simulink model "blovtb"  (Simulink 8.5)
settings: Solver=ode45  SolverMode=SingleTasking  StartTime=0.0  StopTime=6  MaxStep=.002  RelTol=1e-3  AbsTol=1e-6
settings Model: Creator=PC  LastModifiedBy=PC  ExtModeTrigMode=oneshot  ExtModeArmWhenConnect=off
settings DataIOCC: LimitDataPoints=off
settings OptimizationCC: BlockReduction=off  BooleanDataType=off  ExpressionDepthLimit=128
settings DebuggingCC: SaveWithParameterizedLinksMsg=none  SignalResolutionControl=TryResolveAllWithWarning  MultiTaskDSMMsg=warning  MultiTaskCondExecSysMsg=none  FcnCallInpInsideContextMsg=EnableAllAsError  StateNameClashWarn=none  StrictBusMsg=None
settings HardwareCC: TargetUnknown=on

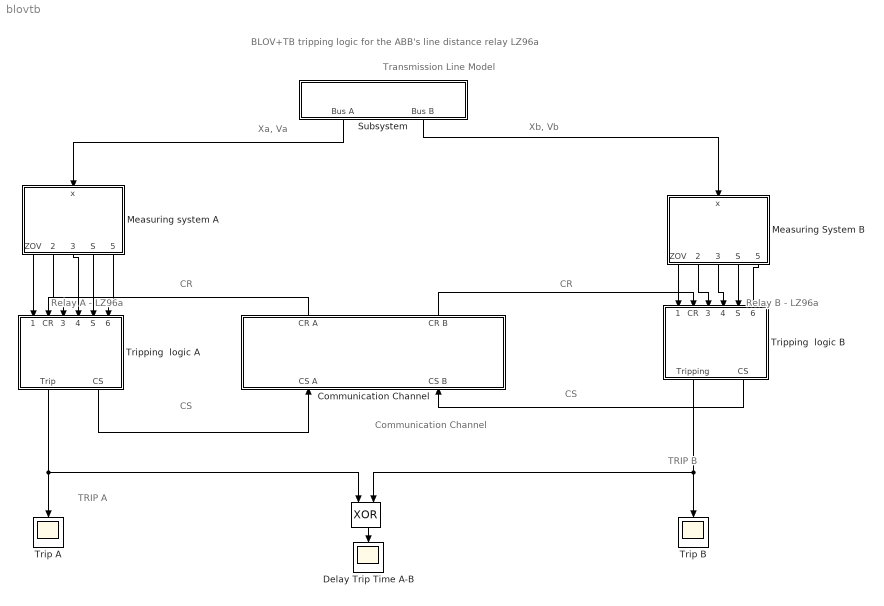
== system blovtb ==
  note: Transmission Line Model
  note: Relay A - LZ96a
  note: Xa, Va
  note: Xb, Vb
  note: CS
  note: CS
  note: CR
  note: CR
  note: TRIP A
  note: TRIP B
  note: Relay B - LZ96a
  note: Communication
      | Channel
  note: BLOV+TB tripping logic for the ABB's line distance relay LZ96a
  " " : Logic  Operator=XOR
  Communication Channel : Subsystem  mask(Communication channel.){Tdelay=0, failureA=on, failureB=on, err_signal=0}
      mask prompts: Tdelay "Channel delay time [ms]:"; failureA "A to B Communication channel failure."; failureB "B to A Communication Channel failure"; err_signal "Erroneous signal:"
      mask TypeOptions err_signal: 0 | 1
  Delay Trip Time A-B : Scope
      settings: TickLabels=on  YMin=-0.5  YMax=2
  Measuring System B : Subsystem  mask(Measuring system - starter block){ZM=[0 1.8 2.5], Tzone=[0 0.4 0.6], S=[-1 3], Tstarter=0.8, ZOV=1.3, ZMB=-1.3, tHF1=0.2}
      mask prompts: ZM "Zone reach [z1 z2  z3]  [p.u.]:"; Tzone "Zone times [z1 z2  z3]  [s]:"; S "Starter range [Smin Smax] [p.u.]:"; Tstarter "Starter time [s]:"; ZOV "ZOV (pu)"; ZMB "ZMB (p.u.):"; tHF1 "tHF(s)"
      mask init:
      | SB=S(1);
      | SF=S(2);
      | t4=Tstarter;
      | ZM1=ZM(1);
      | ZM2=ZM(2);
      | ZM3=ZM(3);
      | t1=Tzone(1);
      | t2=Tzone(2);
      | t3=Tzone(3);
  Measuring system A : Subsystem  mask(Measuring system - starter block){ZM=[0 1.8 2.5], Tzone=[0 0.4 0.6], S=[-1 4], Tstarter=0.8, ZOV=1.3, ZMB=-1.3, tHF1=0.2}
      mask prompts: ZM "Zone reach [z1 z2  z3]  [p.u.]:"; Tzone "Zone times [z1 z2  z3]  [s]:"; S "Starter range [Smin Smax] [p.u.]:"; Tstarter "Starter time [s]:"; ZOV "ZOV (pu)"; ZMB "ZMB (p.u.):"; tHF1 "tHF(s)"
      mask init:
      | SB=S(1);
      | SF=S(2);
      | t4=Tstarter;
      | ZM1=ZM(1);
      | ZM2=ZM(2);
      | ZM3=ZM(3);
      | t1=Tzone(1);
      | t2=Tzone(2);
      | t3=Tzone(3);
  Subsystem : Subsystem  mask(Model of transmission line with fault){x=1.1, Tfault=1}
      mask prompts: x "Fault location from bus A [p.u.]"; Tfault "Fault time [s]:"
  Trip A : Scope
      settings: TickLabels=on  YMin=-0.5  YMax=2
  Trip B : Scope
      settings: TickLabels=on  YMin=-0.5  YMax=2
  Tripping  logic A : Subsystem
  Tripping  logic B : Subsystem
  wires:
  " "/1 -> Delay Trip Time A-B/1
  Measuring system A/4(S) -> Tripping  logic A/5(S)
  Measuring system A/3(ZM3 Output) -> Tripping  logic A/4(ZM3)
  Measuring system A/5(ZMB) -> Tripping  logic A/6(ZMB)
  Subsystem/1(Bus A) -> Measuring system A/1(x)
  Tripping  logic A/2(CS) -> Communication Channel/1(CS A)
  Communication Channel/1(CR A) -> Tripping  logic A/2(CR)
  Measuring System B/4(S) -> Tripping  logic B/5(S)
  Measuring System B/3(ZM3 Output) -> Tripping  logic B/4(ZM3)
  Measuring System B/2(ZM2 Output) -> Tripping  logic B/3(ZM2)
  Measuring System B/5(ZMB) -> Tripping  logic B/6(ZMB)
  Measuring System B/1(ZOV) -> Tripping  logic B/1(ZOV)
  Subsystem/2(Bus B) -> Measuring System B/1(x)
  Tripping  logic B/1(Tripping) -> Trip B/1, " "/2
  Tripping  logic B/2(CS) -> Communication Channel/2(CS B)
  Communication Channel/2(CR B) -> Tripping  logic B/2(CR)
  Tripping  logic A/1(Trip) -> Trip A/1, " "/1
  Measuring system A/1(ZOV) -> Tripping  logic A/1(ZOV)
  Measuring system A/2(ZM2 Output) -> Tripping  logic A/3(ZM2)

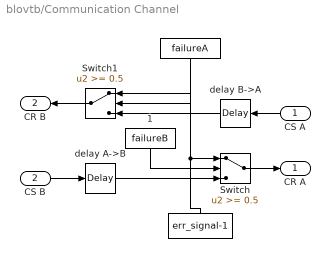
== system blovtb/Communication Channel ==
  CS A : Inport
  CS B : Inport  Port=2
  " " : Constant  Value=failureA
  "  " : Constant  Value=err_signal-1
  " 1" : Constant  Value=failureB
  Switch : Switch  Threshold=0.5  SaturateOnIntegerOverflow=on  InputSameDT=on
  Switch1 : Switch  Threshold=0.5  SaturateOnIntegerOverflow=on  InputSameDT=on
  delay A->B : TransportDelay  DelayTime=Tdelay/1000+1e-12
  delay B->A : TransportDelay  DelayTime=Tdelay/1000+1e-12
  CR A : Outport  InitialOutput=0
  CR B : Outport  Port=2  InitialOutput=0
  wires:
  Switch/1 -> CR A/1
  CS B/1 -> delay A->B/1
  CS A/1 -> delay B->A/1
  Switch1/1 -> CR B/1
  "  "/1 -> Switch1/1, Switch/1
  delay A->B/1 -> Switch/3
  delay B->A/1 -> Switch1/3
  " "/1 -> Switch1/2
  " 1"/1 -> Switch/2

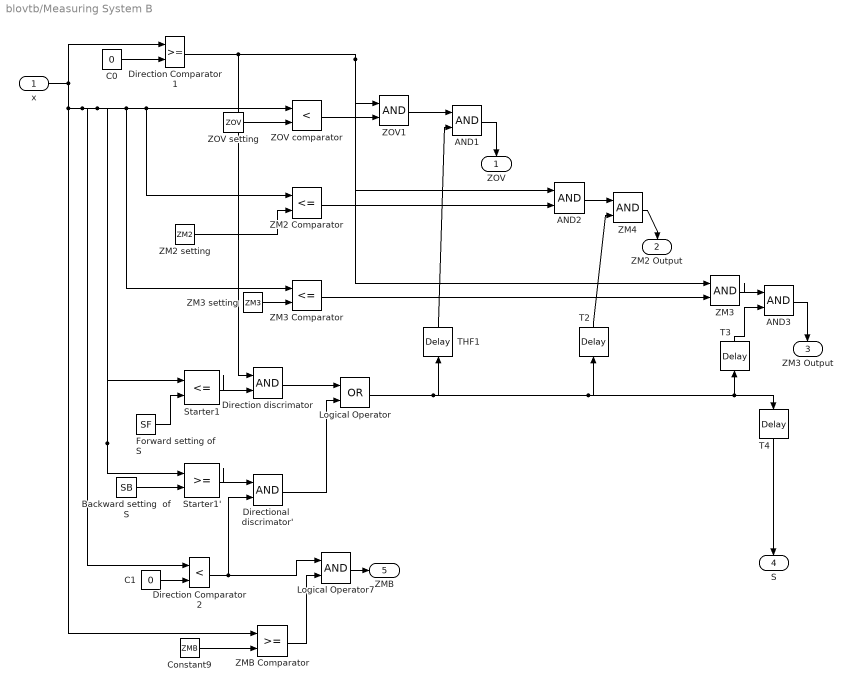
== system blovtb/Measuring System B ==
  x : Inport
  AND1 : Logic
  AND2 : Logic
  AND3 : Logic
  Backward setting  of S : Constant  Value=SB
  C0 : Constant  Value=0
  C1 : Constant  Value=0
  Constant9 : Constant  Value=ZMB
  Direction Comparator1 : RelationalOperator  InputSameDT=on
  Direction Comparator2 : RelationalOperator  Operator=<  InputSameDT=on
  Direction discrimator : Logic
  Directional  discrimator' : Logic
  Forward setting of S : Constant  Value=SF
  Logical Operator : Logic  Operator=OR
  Logical Operator7 : Logic
  Starter1 : RelationalOperator  Operator=<=  InputSameDT=on
  Starter1' : RelationalOperator  InputSameDT=on
  T2 : TransportDelay  DelayTime=t2
  T3 : TransportDelay  DelayTime=t3
  T4 : TransportDelay  DelayTime=t4
  THF1 : TransportDelay  DelayTime=tHF1
  ZM2 Comparator : RelationalOperator  Operator=<=  InputSameDT=on
  ZM2 setting : Constant  Value=ZM2
  ZM3 : Logic
  ZM3 Comparator : RelationalOperator  Operator=<=  InputSameDT=on
  ZM3 setting : Constant  Value=ZM3
  ZM4 : Logic
  ZMB Comparator : RelationalOperator  InputSameDT=on
  ZOV comparator : RelationalOperator  Operator=<  InputSameDT=on
  ZOV setting : Constant  Value=ZOV
  ZOV1 : Logic
  ZOV : Outport  InitialOutput=0
  ZM2 Output : Outport  Port=2  InitialOutput=0
  ZM3 Output : Outport  Port=3  InitialOutput=0
  S : Outport  Port=4  InitialOutput=0
  ZMB : Outport  Port=5  InitialOutput=0
  wires:
  ZM2 setting/1 -> ZM2 Comparator/2
  C0/1 -> Direction Comparator1/2
  x/1 -> Direction Comparator1/1, ZM2 Comparator/1, ZOV comparator/1, ZM3 Comparator/1, Starter1/1, Starter1'/1, Direction Comparator2/1, ZMB Comparator/1
  Forward setting of S/1 -> Starter1/2
  Constant9/1 -> ZMB Comparator/2
  ZMB Comparator/1 -> Logical Operator7/2
  C1/1 -> Direction Comparator2/2
  Logical Operator7/1 -> ZMB/1
  ZM3 Comparator/1 -> ZM3/2
  ZM2 Comparator/1 -> AND2/2
  AND2/1 -> ZM4/1
  ZM3/1 -> AND3/1
  Backward setting  of S/1 -> Starter1'/2
  T4/1 -> S/1
  T2/1 -> ZM4/2
  ZM4/1 -> ZM2 Output/1
  T3/1 -> AND3/2
  AND3/1 -> ZM3 Output/1
  Starter1/1 -> Direction discrimator/2
  Direction Comparator1/1 -> ZOV1/1, AND2/1, ZM3/1, Direction discrimator/1
  Direction discrimator/1 -> Logical Operator/1
  Starter1'/1 -> Directional  discrimator'/1
  Directional  discrimator'/1 -> Logical Operator/2
  Logical Operator/1 -> THF1/1, T2/1, T4/1, T3/1
  Direction Comparator2/1 -> Logical Operator7/1, Directional  discrimator'/2
  ZM3 setting/1 -> ZM3 Comparator/2
  ZOV setting/1 -> ZOV comparator/2
  ZOV comparator/1 -> ZOV1/2
  ZOV1/1 -> AND1/1
  THF1/1 -> AND1/2
  AND1/1 -> ZOV/1

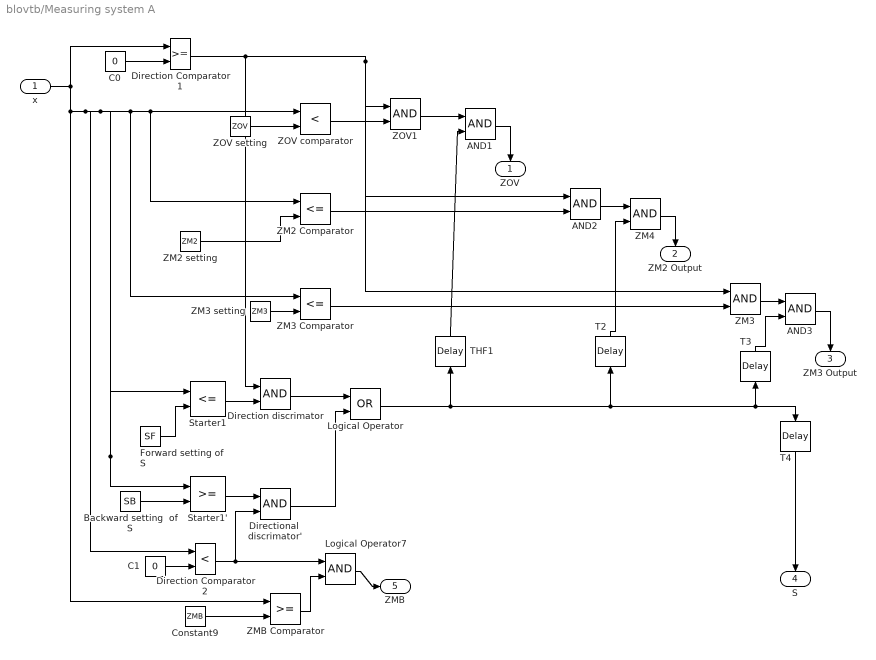
== system blovtb/Measuring system A ==
  x : Inport
  AND1 : Logic
  AND2 : Logic
  AND3 : Logic
  Backward setting  of S : Constant  Value=SB
  C0 : Constant  Value=0
  C1 : Constant  Value=0
  Constant9 : Constant  Value=ZMB
  Direction Comparator1 : RelationalOperator  InputSameDT=on
  Direction Comparator2 : RelationalOperator  Operator=<  InputSameDT=on
  Direction discrimator : Logic
  Directional  discrimator' : Logic
  Forward setting of S : Constant  Value=SF
  Logical Operator : Logic  Operator=OR
  Logical Operator7 : Logic
  Starter1 : RelationalOperator  Operator=<=  InputSameDT=on
  Starter1' : RelationalOperator  InputSameDT=on
  T2 : TransportDelay  DelayTime=t2
  T3 : TransportDelay  DelayTime=t3
  T4 : TransportDelay  DelayTime=t4
  THF1 : TransportDelay  DelayTime=tHF1
  ZM2 Comparator : RelationalOperator  Operator=<=  InputSameDT=on
  ZM2 setting : Constant  Value=ZM2
  ZM3 : Logic
  ZM3 Comparator : RelationalOperator  Operator=<=  InputSameDT=on
  ZM3 setting : Constant  Value=ZM3
  ZM4 : Logic
  ZMB Comparator : RelationalOperator  InputSameDT=on
  ZOV comparator : RelationalOperator  Operator=<  InputSameDT=on
  ZOV setting : Constant  Value=ZOV
  ZOV1 : Logic
  ZOV : Outport  InitialOutput=0
  ZM2 Output : Outport  Port=2  InitialOutput=0
  ZM3 Output : Outport  Port=3  InitialOutput=0
  S : Outport  Port=4  InitialOutput=0
  ZMB : Outport  Port=5  InitialOutput=0
  wires:
  ZM2 setting/1 -> ZM2 Comparator/2
  C0/1 -> Direction Comparator1/2
  x/1 -> Direction Comparator1/1, ZM2 Comparator/1, ZOV comparator/1, ZM3 Comparator/1, Starter1/1, Starter1'/1, Direction Comparator2/1, ZMB Comparator/1
  Forward setting of S/1 -> Starter1/2
  Constant9/1 -> ZMB Comparator/2
  ZMB Comparator/1 -> Logical Operator7/2
  C1/1 -> Direction Comparator2/2
  Logical Operator7/1 -> ZMB/1
  ZM3 Comparator/1 -> ZM3/2
  ZM2 Comparator/1 -> AND2/2
  AND2/1 -> ZM4/1
  ZM3/1 -> AND3/1
  Backward setting  of S/1 -> Starter1'/2
  T4/1 -> S/1
  T2/1 -> ZM4/2
  ZM4/1 -> ZM2 Output/1
  T3/1 -> AND3/2
  AND3/1 -> ZM3 Output/1
  Starter1/1 -> Direction discrimator/2
  Direction Comparator1/1 -> ZOV1/1, AND2/1, ZM3/1, Direction discrimator/1
  Direction discrimator/1 -> Logical Operator/1
  Starter1'/1 -> Directional  discrimator'/1
  Directional  discrimator'/1 -> Logical Operator/2
  Logical Operator/1 -> THF1/1, T2/1, T4/1, T3/1
  Direction Comparator2/1 -> Logical Operator7/1, Directional  discrimator'/2
  ZM3 setting/1 -> ZM3 Comparator/2
  ZOV setting/1 -> ZOV comparator/2
  ZOV comparator/1 -> ZOV1/2
  ZOV1/1 -> AND1/1
  THF1/1 -> AND1/2
  AND1/1 -> ZOV/1

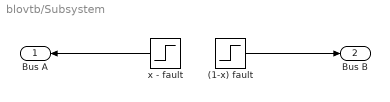
== system blovtb/Subsystem ==
  (1-x) fault : Step  Time=Tfault  Before=1000  After=1-x  SampleTime=0
  x - fault : Step  Time=Tfault  Before=1000  After=x  SampleTime=0
  Bus A : Outport  InitialOutput=0
  Bus B : Outport  Port=2  InitialOutput=0
  wires:
  x - fault/1 -> Bus A/1
  (1-x) fault/1 -> Bus B/1

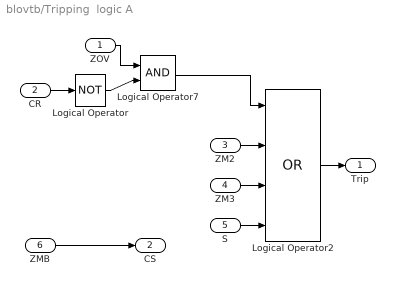
== system blovtb/Tripping  logic A ==
  ZOV : Inport
  CR : Inport  Port=2
  ZM2 : Inport  Port=3
  ZM3 : Inport  Port=4
  S : Inport  Port=5
  ZMB : Inport  Port=6
  Logical Operator : Logic  Operator=NOT  Inputs=1
  Logical Operator2 : Logic  Operator=OR  Inputs=4
  Logical Operator7 : Logic
  Trip : Outport  InitialOutput=0
  CS : Outport  Port=2  InitialOutput=0
  wires:
  ZMB/1 -> CS/1
  S/1 -> Logical Operator2/4
  ZM3/1 -> Logical Operator2/3
  Logical Operator2/1 -> Trip/1
  ZM2/1 -> Logical Operator2/2
  CR/1 -> Logical Operator/1
  ZOV/1 -> Logical Operator7/1
  Logical Operator/1 -> Logical Operator7/2
  Logical Operator7/1 -> Logical Operator2/1

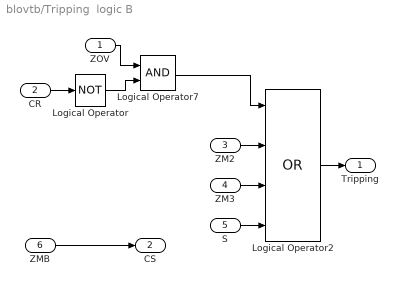
== system blovtb/Tripping  logic B ==
  ZOV : Inport
  CR : Inport  Port=2
  ZM2 : Inport  Port=3
  ZM3 : Inport  Port=4
  S : Inport  Port=5
  ZMB : Inport  Port=6
  Logical Operator : Logic  Operator=NOT  Inputs=1
  Logical Operator2 : Logic  Operator=OR  Inputs=4
  Logical Operator7 : Logic
  Tripping : Outport  InitialOutput=0
  CS : Outport  Port=2  InitialOutput=0
  wires:
  ZMB/1 -> CS/1
  S/1 -> Logical Operator2/4
  ZM3/1 -> Logical Operator2/3
  Logical Operator2/1 -> Tripping/1
  ZM2/1 -> Logical Operator2/2
  CR/1 -> Logical Operator/1
  ZOV/1 -> Logical Operator7/1
  Logical Operator/1 -> Logical Operator7/2
  Logical Operator7/1 -> Logical Operator2/1
